simulink model "Basic_DMT"  (R2014b)
settings: Solver=FixedStepDiscrete  SolverMode=SingleTasking  StartTime=0.0  StopTime=25e-6-14e-9*24  RelTol=1e-3
PreLoadFcn:
  | userName = getenv('UserName');
  | 
  | if strcmp(userName,'Tim')
  | cd C:\Users\Tim\Documents\GitHub\MA_1\Basic_DMT
  | else
  | cd C:\Users\Tim-UML\Documents\GitHub\MA_1\Basic_DMT
  | end
InitFcn:
  | userName = getenv('UserName');
  | 
  | if strcmp(userName,'Tim')
  | cd C:\Users\Tim\Documents\GitHub\MA_1\Basic_DMT
  | else
  | cd C:\Users\Tim-UML\Documents\GitHub\MA_1\Basic_DMT
  | end
values from neighbouring files (symbols this model uses):
  a0 = 0.21194908595403703    (= 0.211949085954)    [initScript.m]
  a1 = 0.576101828091926    (= 0.576101828092)    [initScript.m]
  a2 = a0    (= 0.211949085954)    [initScript.m]
  beta = 1    [initScript.m]
  bitPerSymb = 4    [initScript.m]
  chanDownFact = Tchan/SystemPeriod    [initScript.m]
  fftLen = 16    [initScript.m]
  fftLenActive = fftLenDMT    (= 32)    [initScript.m]
  fftLenDMT = 2*fftLen    (= 32)    [initScript.m]
  GI_Active = GI_LenDMT    (= 0)    [initScript.m]
  GI_Len = 0    [initScript.m]
  GI_LenDMT = 0    [initScript.m]
  M = log2(fftLen)    [initScript.m]
  sysgenSystemPeriod = 4e-9    (= 4e-09)    [initScript.m]
  SystemPeriod = 4e-9    (= 4e-09)    [initScript.m]
  upsampleFactor = 1    [initScript.m]
  usedSubCar = 14    [initScript.m]
undefined symbols (not defined in the file or in its folder): bitCount, get, modu_mode, Tb, Ts
libraries: xbsIndex_r4 x822, commdigbbndam3 x59, simulink x42, dspsigops x7, commrandsrc2 x6, dspbuff3 x4, dspxfrm3 x3, dspswit3 x2, commseqgen2 x1, dsparch4 x1, commutil2 x1, dspsnks4 x1
(part 4 of 10)

== system Basic_DMT/Demodulation/Bit Demapping P11 ==
  mode : Inport
  data : Inport  Port=2
  16-QAM : Subsystem
  256-QAM : Subsystem
  Fcn : Fcn  Expr=u==0
  Fcn1 : Fcn  Expr=u==1
  Merge : Merge
  Out1 : Outport
  wires:
  data/1 -> 16-QAM/1(In1), 256-QAM/1(In1)
  Fcn/1 -> 256-QAM/Enable
  mode/1 -> Fcn1/1, Fcn/1
  Merge/1 -> Out1/1
  Fcn1/1 -> 16-QAM/Enable
  256-QAM/1(Out1) -> Merge/2
  16-QAM/1(Out1) -> Merge/1

== system Basic_DMT/Demodulation/Bit Demapping P12 ==
  mode : Inport
  data : Inport  Port=2
  16-QAM : Subsystem
  256-QAM : Subsystem
  Fcn : Fcn  Expr=u==0
  Fcn1 : Fcn  Expr=u==1
  Merge : Merge
  Out1 : Outport
  wires:
  data/1 -> 16-QAM/1(In1), 256-QAM/1(In1)
  Fcn/1 -> 256-QAM/Enable
  mode/1 -> Fcn1/1, Fcn/1
  Merge/1 -> Out1/1
  Fcn1/1 -> 16-QAM/Enable
  256-QAM/1(Out1) -> Merge/2
  16-QAM/1(Out1) -> Merge/1

== system Basic_DMT/Demodulation/Bit Demapping P13 ==
  mode : Inport
  data : Inport  Port=2
  16-QAM : Subsystem
  256-QAM : Subsystem
  Fcn : Fcn  Expr=u==0
  Fcn1 : Fcn  Expr=u==1
  Merge : Merge
  Out1 : Outport
  wires:
  data/1 -> 16-QAM/1(In1), 256-QAM/1(In1)
  Fcn/1 -> 256-QAM/Enable
  mode/1 -> Fcn1/1, Fcn/1
  Merge/1 -> Out1/1
  Fcn1/1 -> 16-QAM/Enable
  256-QAM/1(Out1) -> Merge/2
  16-QAM/1(Out1) -> Merge/1

== system Basic_DMT/Demodulation/Bit Demapping P14 ==
  mode : Inport
  data : Inport  Port=2
  16-QAM : Subsystem
  256-QAM : Subsystem
  Fcn : Fcn  Expr=u==0
  Fcn1 : Fcn  Expr=u==1
  Merge : Merge
  Out1 : Outport
  wires:
  data/1 -> 16-QAM/1(In1), 256-QAM/1(In1)
  Fcn/1 -> 256-QAM/Enable
  mode/1 -> Fcn1/1, Fcn/1
  Merge/1 -> Out1/1
  Fcn1/1 -> 16-QAM/Enable
  256-QAM/1(Out1) -> Merge/2
  16-QAM/1(Out1) -> Merge/1

== system Basic_DMT/Demodulation/Bit Demapping P2 ==
  mode : Inport
  data : Inport  Port=2
  16-QAM : Subsystem
  256-QAM : Subsystem
  Fcn : Fcn  Expr=u==0
  Fcn1 : Fcn  Expr=u==1
  Merge : Merge
  Out1 : Outport
  wires:
  data/1 -> 16-QAM/1(In1), 256-QAM/1(In1)
  Fcn/1 -> 256-QAM/Enable
  mode/1 -> Fcn1/1, Fcn/1
  Merge/1 -> Out1/1
  Fcn1/1 -> 16-QAM/Enable
  256-QAM/1(Out1) -> Merge/2
  16-QAM/1(Out1) -> Merge/1

== system Basic_DMT/Demodulation/Bit Demapping P3 ==
  mode : Inport
  data : Inport  Port=2
  16-QAM : Subsystem
  256-QAM : Subsystem
  Fcn : Fcn  Expr=u==0
  Fcn1 : Fcn  Expr=u==1
  Merge : Merge
  Out1 : Outport
  wires:
  data/1 -> 16-QAM/1(In1), 256-QAM/1(In1)
  Fcn/1 -> 256-QAM/Enable
  mode/1 -> Fcn1/1, Fcn/1
  Merge/1 -> Out1/1
  Fcn1/1 -> 16-QAM/Enable
  256-QAM/1(Out1) -> Merge/2
  16-QAM/1(Out1) -> Merge/1

== system Basic_DMT/Demodulation/Bit Demapping P4 ==
  mode : Inport
  data : Inport  Port=2
  16-QAM : Subsystem
  256-QAM : Subsystem
  Fcn : Fcn  Expr=u==0
  Fcn1 : Fcn  Expr=u==1
  Merge : Merge
  Out1 : Outport
  wires:
  data/1 -> 16-QAM/1(In1), 256-QAM/1(In1)
  Fcn/1 -> 256-QAM/Enable
  mode/1 -> Fcn1/1, Fcn/1
  Merge/1 -> Out1/1
  Fcn1/1 -> 16-QAM/Enable
  256-QAM/1(Out1) -> Merge/2
  16-QAM/1(Out1) -> Merge/1

== system Basic_DMT/Demodulation/Bit Demapping P5 ==
  mode : Inport
  data : Inport  Port=2
  16-QAM : Subsystem
  256-QAM : Subsystem
  Fcn : Fcn  Expr=u==0
  Fcn1 : Fcn  Expr=u==1
  Merge : Merge
  Out1 : Outport
  wires:
  data/1 -> 16-QAM/1(In1), 256-QAM/1(In1)
  Fcn/1 -> 256-QAM/Enable
  mode/1 -> Fcn1/1, Fcn/1
  Merge/1 -> Out1/1
  Fcn1/1 -> 16-QAM/Enable
  256-QAM/1(Out1) -> Merge/2
  16-QAM/1(Out1) -> Merge/1

== system Basic_DMT/Demodulation/Bit Demapping P6 ==
  mode : Inport
  data : Inport  Port=2
  16-QAM : Subsystem
  256-QAM : Subsystem
  Fcn : Fcn  Expr=u==0
  Fcn1 : Fcn  Expr=u==1
  Merge : Merge
  Out1 : Outport
  wires:
  data/1 -> 16-QAM/1(In1), 256-QAM/1(In1)
  Fcn/1 -> 256-QAM/Enable
  mode/1 -> Fcn1/1, Fcn/1
  Merge/1 -> Out1/1
  Fcn1/1 -> 16-QAM/Enable
  256-QAM/1(Out1) -> Merge/2
  16-QAM/1(Out1) -> Merge/1

== system Basic_DMT/Demodulation/Bit Demapping P7 ==
  mode : Inport
  data : Inport  Port=2
  16-QAM : Subsystem
  256-QAM : Subsystem
  Fcn : Fcn  Expr=u==0
  Fcn1 : Fcn  Expr=u==1
  Merge : Merge
  Out1 : Outport
  wires:
  data/1 -> 16-QAM/1(In1), 256-QAM/1(In1)
  Fcn/1 -> 256-QAM/Enable
  mode/1 -> Fcn1/1, Fcn/1
  Merge/1 -> Out1/1
  Fcn1/1 -> 16-QAM/Enable
  256-QAM/1(Out1) -> Merge/2
  16-QAM/1(Out1) -> Merge/1

== system Basic_DMT/Demodulation/Bit Demapping P8 ==
  mode : Inport
  data : Inport  Port=2
  16-QAM : Subsystem
  256-QAM : Subsystem
  Fcn : Fcn  Expr=u==0
  Fcn1 : Fcn  Expr=u==1
  Merge : Merge
  Out1 : Outport
  wires:
  data/1 -> 16-QAM/1(In1), 256-QAM/1(In1)
  Fcn/1 -> 256-QAM/Enable
  mode/1 -> Fcn1/1, Fcn/1
  Merge/1 -> Out1/1
  Fcn1/1 -> 16-QAM/Enable
  256-QAM/1(Out1) -> Merge/2
  16-QAM/1(Out1) -> Merge/1

== system Basic_DMT/Demodulation/Bit Demapping P9 ==
  mode : Inport
  data : Inport  Port=2
  16-QAM : Subsystem
  256-QAM : Subsystem
  Fcn : Fcn  Expr=u==0
  Fcn1 : Fcn  Expr=u==1
  Merge : Merge
  Out1 : Outport
  wires:
  data/1 -> 16-QAM/1(In1), 256-QAM/1(In1)
  Fcn/1 -> 256-QAM/Enable
  mode/1 -> Fcn1/1, Fcn/1
  Merge/1 -> Out1/1
  Fcn1/1 -> 16-QAM/Enable
  256-QAM/1(Out1) -> Merge/2
  16-QAM/1(Out1) -> Merge/1

== system Basic_DMT/IFFTaPIS/Assert_After_Create_Frame ==
  In1 : Inport
  In2 : Inport  Port=2
  In3 : Inport  Port=3
  Add1 : Sum  Inputs=+-
  Add3 : Sum  Inputs=+-
  Check Static Range1 : simulink/Model Verification/Check  Static Range  Description=0 <= u <= 0  max=0  max_included=on  min=0  min_included=on  enabled=on  stopWhenAssertionFail=off  export=off  icon=graphic
  Check Static Range3 : simulink/Model Verification/Check  Static Range  Description=0 <= u <= 0  max=0  max_included=on  min=0  min_included=on  enabled=on  stopWhenAssertionFail=off  export=off  icon=graphic
  Complex to Real-Imag : ComplexToRealImag
  Delay : Delay  DelayLength=1  InitialCondition=0
  Gateway Out6 : xbsIndex_r4/Gateway Out  inherit_from_input=off  hdl_port=off  rows=1  columns=1  UseAsDAC=off  DACChannel='1'  interface=None  automatic_assignment=on  address_offset=hex2dec('00')  intf_description=''  timing_constraint=None  locs_specified=off  LOCs={}  io_standard={}  block_type=gatewayout
  Gateway Out7 : xbsIndex_r4/Gateway Out  inherit_from_input=off  hdl_port=off  rows=1  columns=1  UseAsDAC=off  DACChannel='1'  interface=None  automatic_assignment=on  address_offset=hex2dec('00')  intf_description=''  timing_constraint=None  locs_specified=off  LOCs={}  io_standard={}  block_type=gatewayout
  Scope1 : Scope  NumInputPorts=6
      settings: TimeRange=4.014342186534899e-07  YMin=-3~-3~-4~-4~-4~-10  YMax=1~1~4~4~4~10  SaveName=ScopeData24
  Unbuffer2 : Unbuffer  SampleBasedProcessing=Same as frame based
  wires:
  In2/1 -> Gateway Out6/1
  In3/1 -> Gateway Out7/1
  Complex to Real-Imag/1 -> Scope1/1, Add3/1
  Gateway Out6/1 -> Scope1/2, Add3/2
  Add3/1 -> Scope1/3, Check Static Range3/1
  Gateway Out7/1 -> Scope1/5, Add1/2
  Complex to Real-Imag/2 -> Scope1/4, Add1/1
  Add1/1 -> Scope1/6, Check Static Range1/1
  Unbuffer2/1 -> Delay/1
  Delay/1 -> Complex to Real-Imag/1
  In1/1 -> Unbuffer2/1

== system Basic_DMT/IFFTaPIS/Assert_After_IFFT ==
  In1 : Inport
  In2 : Inport  Port=2
  In3 : Inport  Port=3
  Add1 : Sum  Inputs=+-
  Add3 : Sum  Inputs=+-
  Check Static Range1 : simulink/Model Verification/Check  Static Range  Description=0 <= u <= 0  max=0  max_included=on  min=0  min_included=on  enabled=on  stopWhenAssertionFail=off  export=off  icon=graphic
  Check Static Range3 : simulink/Model Verification/Check  Static Range  Description=0 <= u <= 0  max=0  max_included=on  min=0  min_included=on  enabled=on  stopWhenAssertionFail=off  export=off  icon=graphic
  Complex to Real-Imag : ComplexToRealImag
  Delay : Delay  Commented=through  DelayLength=1  InitialCondition=0
  Gateway Out6 : xbsIndex_r4/Gateway Out  inherit_from_input=off  hdl_port=off  rows=1  columns=1  UseAsDAC=off  DACChannel='1'  interface=None  automatic_assignment=on  address_offset=hex2dec('00')  intf_description=''  timing_constraint=None  locs_specified=off  LOCs={}  io_standard={}  block_type=gatewayout
  Gateway Out7 : xbsIndex_r4/Gateway Out  inherit_from_input=off  hdl_port=off  rows=1  columns=1  UseAsDAC=off  DACChannel='1'  interface=None  automatic_assignment=on  address_offset=hex2dec('00')  intf_description=''  timing_constraint=None  locs_specified=off  LOCs={}  io_standard={}  block_type=gatewayout
  Scope1 : Scope  NumInputPorts=6
      settings: YMin=-5~-5~-5~-5~-5~-5  YMax=5~5~5~5~5~5  SaveName=ScopeData24
  Unbuffer2 : Unbuffer  SampleBasedProcessing=Same as frame based
  wires:
  In2/1 -> Gateway Out6/1
  In3/1 -> Gateway Out7/1
  Complex to Real-Imag/1 -> Scope1/1, Add3/1
  Gateway Out6/1 -> Add3/2, Scope1/2
  Add3/1 -> Check Static Range3/1, Scope1/3
  Gateway Out7/1 -> Add1/2, Scope1/5
  Complex to Real-Imag/2 -> Add1/1, Scope1/4
  Add1/1 -> Check Static Range1/1, Scope1/6
  Unbuffer2/1 -> Delay/1
  Delay/1 -> Complex to Real-Imag/1
  In1/1 -> Unbuffer2/1

== system Basic_DMT/IFFTaPIS/Assert_aft_GI ==
  In1 : Inport
  In2 : Inport  Port=2
  In3 : Inport  Port=3
  Abs{,1..5} (6 alike) : Abs
  Add1 : Sum  Inputs=+-
  Add2 : Sum  Inputs=+-
  Add3 : Sum  Inputs=+-
  Complex to Real-Imag : ComplexToRealImag
  Data Type Conversion1 : DataTypeConversion  OutDataTypeStr=double
  Data Type Conversion2 : DataTypeConversion  OutDataTypeStr=double
  Delay : Delay  Commented=through  DelayLength=62  InitialCondition=0
  Divide : Product  Inputs=*/
  Divide1 : Product  Inputs=*/
  Divide2 : Product  Inputs=*/
  Gateway Out6 : xbsIndex_r4/Gateway Out  inherit_from_input=off  hdl_port=off  rows=1  columns=1  UseAsDAC=off  DACChannel='1'  interface=None  automatic_assignment=on  address_offset=hex2dec('00')  intf_description=''  timing_constraint=None  locs_specified=off  LOCs={}  io_standard={}  block_type=gatewayout
  Gateway Out7 : xbsIndex_r4/Gateway Out  inherit_from_input=off  hdl_port=off  rows=1  columns=1  UseAsDAC=off  DACChannel='1'  interface=None  automatic_assignment=on  address_offset=hex2dec('00')  intf_description=''  timing_constraint=None  locs_specified=off  LOCs={}  io_standard={}  block_type=gatewayout
  MinMax : MinMax  Function=max  Inputs=2
  MinMax1 : MinMax  Function=max  Inputs=2
  MinMax2 : MinMax  Function=max  Inputs=2
  Real-Imag to Complex : RealImagToComplex
  Scope1 : Scope  Commented=on  NumInputPorts=4
      settings: YMin=-5~-5~-5~-5  YMax=5~5~5~5  SaveName=ScopeData23
  Scope10 : Scope  NumInputPorts=4
      settings: TimeRange=5e-05  YMin=-5~-5~-5~-5  YMax=5~5~5~5  SaveName=ScopeData20
  Scope3 : Scope  Commented=on  NumInputPorts=4
      settings: TimeRange=5e-05  YMin=-5~-5~-5~-5  YMax=5~5~5~5  SaveName=ScopeData21
  wires:
  Data Type Conversion2/1 -> Abs1/1
  Add1/1 -> Scope10/3, Divide/1
  In1/1 -> Delay/1
  Complex to Real-Imag/1 -> Add1/1, Abs3/1, Scope10/1
  In3/1 -> Gateway Out7/1
  In2/1 -> Gateway Out6/1
  Abs/1 -> MinMax2/2, Add3/2, Scope1/2
  Add3/1 -> Divide2/1, Scope1/3
  Abs1/1 -> Scope1/1, MinMax2/1, Add3/1
  Gateway Out6/1 -> Real-Imag to Complex/1, Add1/2, Abs2/1, Scope10/2
  Data Type Conversion1/1 -> Abs/1
  Real-Imag to Complex/1 -> Data Type Conversion1/1
  Delay/1 -> Data Type Conversion2/1, Complex to Real-Imag/1
  MinMax/1 -> Divide/2
  Divide/1 -> Scope10/4
  Add2/1 -> Divide1/1, Scope3/3
  Complex to Real-Imag/2 -> Abs4/1, Scope3/1, Add2/1
  Gateway Out7/1 -> Real-Imag to Complex/2, Abs5/1, Scope3/2, Add2/2
  MinMax1/1 -> Divide1/2
  Divide1/1 -> Scope3/4
  Divide2/1 -> Scope1/4
  MinMax2/1 -> Divide2/2
  Abs2/1 -> MinMax/2
  Abs3/1 -> MinMax/1
  Abs4/1 -> MinMax1/1
  Abs5/1 -> MinMax1/2

== system Basic_DMT/IFFTaPIS/Create_Frame_for_IFFT ==
  note: Unbuffer necessary,
      |  because of frame based signal
  Sub1 : Inport
  Sub2 : Inport  Port=2
  Sub3 : Inport  Port=3
  Sub4 : Inport  Port=4
  Sub5 : Inport  Port=5
  Sub6 : Inport  Port=6
  Sub7 : Inport  Port=7
  Sub8 : Inport  Port=8
  Sub9 : Inport  Port=9
  Sub10 : Inport  Port=10
  Sub11 : Inport  Port=11
  Sub12 : Inport  Port=12
  Sub13 : Inport  Port=13
  Sub14 : Inport  Port=14
  OFDMorDMT : Subsystem  Variant=on
  Unbuffer{1..14} (14 alike) : Unbuffer  SampleBasedProcessing=Same as frame based
  Out1 : Outport
  wires:
  Sub2/1 -> Unbuffer2/1
  Sub1/1 -> Unbuffer3/1
  Unbuffer2/1 -> OFDMorDMT/2(Sub2)
  Unbuffer3/1 -> OFDMorDMT/1(Sub1)
  OFDMorDMT/1(Out1) -> Out1/1
  Sub4/1 -> Unbuffer1/1
  Sub3/1 -> Unbuffer4/1
  Unbuffer1/1 -> OFDMorDMT/4(Sub4)
  Unbuffer4/1 -> OFDMorDMT/3(Sub3)
  Sub6/1 -> Unbuffer5/1
  Sub5/1 -> Unbuffer6/1
  Unbuffer5/1 -> OFDMorDMT/6(Sub6)
  Unbuffer6/1 -> OFDMorDMT/5(Sub5)
  Sub8/1 -> Unbuffer7/1
  Sub7/1 -> Unbuffer8/1
  Unbuffer7/1 -> OFDMorDMT/8(Sub8)
  Unbuffer8/1 -> OFDMorDMT/7(Sub7)
  Sub10/1 -> Unbuffer9/1
  Sub9/1 -> Unbuffer10/1
  Unbuffer9/1 -> OFDMorDMT/10(Sub10)
  Unbuffer10/1 -> OFDMorDMT/9(Sub9)
  Sub11/1 -> Unbuffer11/1
  Unbuffer11/1 -> OFDMorDMT/11(Sub11)
  Sub13/1 -> Unbuffer14/1
  Unbuffer14/1 -> OFDMorDMT/13(Sub13)
  Sub14/1 -> Unbuffer13/1
  Unbuffer13/1 -> OFDMorDMT/14(Sub14)
  Sub12/1 -> Unbuffer12/1
  Unbuffer12/1 -> OFDMorDMT/12(Sub12)

== system Basic_DMT/IFFTaPIS/FSM_FIFO ==
  In1 : Inport  SampleTime=bitPerSymb*usedSubCar*SystemPeriod
  Buffer : Buffer  N=fftLenActive  TreatMby1Signals=One channel
  Complex to Real-Imag{,1..3} (4 alike) : ComplexToRealImag
  Constant2 : Constant  Value=0  SampleTime=SystemPeriod
  Data Store Memory3 : DataStoreMemory  DataStoreName=state  OutDataTypeStr=double
  Data Store Memory4 : DataStoreMemory  DataStoreName=k  OutDataTypeStr=double
  Data Store Memory5 : DataStoreMemory  DataStoreName=loopCount  OutDataTypeStr=double
  Delay : Delay  DelayLength=1  InitialCondition=0
  Index Vector : MultiPortSwitch  DataPortOrder=Zero-based contiguous  Inputs=2  zeroidx=on
  MATLAB Function1 : MATLAB Function  TreatAsAtomicUnit=on  SystemSampleTime=SystemPeriod
  Queue1 : dspbuff3/Queue  depth=64  trigger=Non-zero sample  overflow=Dynamic reallocation  pes=Warning  eso=off  fso=off  nso=on  clr=off  clrOutport=off  adf=off
  Real-Imag to Complex1 : RealImagToComplex
  Scope : Scope  NumInputPorts=2
      settings: YMin=-5~-5  YMax=5~5  SaveName=ScopeData77
  Scope1 : Scope  NumInputPorts=2
      settings: YMin=-5~-5  YMax=5~5  SaveName=ScopeData78
  Unbuffer1 : Unbuffer  ic=64e-9  SampleBasedProcessing=Same as frame based
  Unbuffer2 : Unbuffer  ic=64e-9  SampleBasedProcessing=Same as frame based
  Zero-Order Hold : ZeroOrderHold  SampleTime=SystemPeriod
  Zero-Order Hold1 : ZeroOrderHold  SampleTime=SystemPeriod*16
  Out1 : Outport
  wires:
  Index Vector/1 -> Buffer/1
  MATLAB Function1/3(pop) -> Queue1/3
  MATLAB Function1/2(push) -> Queue1/2
  Constant2/1 -> Real-Imag to Complex1/2, Real-Imag to Complex1/1
  Delay/1 -> MATLAB Function1/1(num)
  MATLAB Function1/1(sel) -> Index Vector/1
  Queue1/1 -> Index Vector/3
  Real-Imag to Complex1/1 -> Index Vector/2
  Buffer/1 -> Out1/1
  Queue1/2 -> Delay/1
  Zero-Order Hold/1 -> Complex to Real-Imag1/1, Queue1/1
  Unbuffer2/1 -> Complex to Real-Imag2/1, Complex to Real-Imag/1, Zero-Order Hold/1
  Complex to Real-Imag/1 -> Scope/1
  Complex to Real-Imag1/1 -> Scope/2
  Zero-Order Hold1/1 -> Unbuffer1/1
  Unbuffer1/1 -> Complex to Real-Imag3/1
  In1/1 -> Zero-Order Hold1/1, Unbuffer2/1
  Complex to Real-Imag2/1 -> Scope1/1
  Complex to Real-Imag3/1 -> Scope1/2

== system Basic_DMT/IFFTaPIS/Guard_Interval ==
  note: 1) Add Subsystem or Model blocks as valid variant choices.
      | 2) You cannot connect blocks at this level. At simulation, connectivity is automatically
      | determined, based on the active variant and port name matching.
  In1 : Inport
  None : Subsystem  VariantControl=guardInterval==1
  Set_GI_DMT : Subsystem  VariantControl=guardInterval==2&&dmtOfdm==2
  Set_GI_OFDM : Subsystem  VariantControl=guardInterval==2&&dmtOfdm==1
  Out1 : Outport
  pop : Outport  Port=2

== system Basic_DMT/IFFTaPIS/upsample ==
  note: 1) Add Subsystem or Model blocks as valid variant choices.
      | 2) You cannot connect blocks at this level. At simulation, connectivity is automatically
      | determined, based on the active variant and port name matching.
  In1 : Inport
  upsample_No : Subsystem  VariantControl=upsample==1
  upsample_yes : Subsystem  VariantControl=upsample==2
  Out1 : Outport

== system Basic_DMT/Modulation/Assert_aft_Mapping ==
  Sub1 : Inport
  Sub2 : Inport  Port=2
  sg_sub1_re : Inport  Port=3
  sg_sub1_im : Inport  Port=4
  sg_sub2_re : Inport  Port=5
  sg_sub2_im : Inport  Port=6
  Add{1..4} (4 alike) : Sum  Inputs=+-
  Check Static Range{1..4} (4 alike) : simulink/Model Verification/Check  Static Range  Description=0 <= u <= 0  max=0  max_included=on  min=0  min_included=on  enabled=on  stopWhenAssertionFail=off  export=off  icon=graphic
  Complex to Real-Imag : ComplexToRealImag
  Complex to Real-Imag1 : ComplexToRealImag
  Gateway Out{1..2,6..7} (4 alike) : xbsIndex_r4/Gateway Out  inherit_from_input=off  hdl_port=off  rows=1  columns=1  UseAsDAC=off  DACChannel='1'  interface=None  automatic_assignment=on  address_offset=hex2dec('00')  intf_description=''  timing_constraint=None  locs_specified=off  LOCs={}  io_standard={}  block_type=gatewayout
  Scope{1..3,10} (4 alike) : Scope  Commented=on  NumInputPorts=3
      Scope1 settings: YMin=-5~-5~-5  YMax=5~5~5  SaveName=ScopeData25
      Scope10 settings: YMin=-5~-5~-5  YMax=5~5~5  SaveName=ScopeData14
      Scope2 settings: YMin=-5~-5~-5  YMax=5~5~5  SaveName=ScopeData26
      Scope3 settings: YMin=-5~-5~-5  YMax=5~5~5  SaveName=ScopeData8
  wires:
  Gateway Out7/1 -> Scope3/2, Add2/2
  Add1/1 -> Check Static Range2/1, Scope10/3
  Gateway Out6/1 -> Scope10/2, Add1/2
  Complex to Real-Imag/2 -> Scope3/1, Add2/1
  Complex to Real-Imag/1 -> Add1/1, Scope10/1
  Sub1/1 -> Complex to Real-Imag/1
  Add2/1 -> Check Static Range1/1, Scope3/3
  sg_sub1_re/1 -> Gateway Out6/1
  sg_sub1_im/1 -> Gateway Out7/1
  sg_sub2_re/1 -> Gateway Out1/1
  sg_sub2_im/1 -> Gateway Out2/1
  Gateway Out2/1 -> Scope2/2, Add4/2
  Add3/1 -> Check Static Range4/1, Scope1/3
  Gateway Out1/1 -> Scope1/2, Add3/2
  Complex to Real-Imag1/2 -> Scope2/1, Add4/1
  Complex to Real-Imag1/1 -> Add3/1, Scope1/1
  Add4/1 -> Check Static Range3/1, Scope2/3
  Sub2/1 -> Complex to Real-Imag1/1

== system Basic_DMT/Modulation/Bit_Mapping_P1 ==
  mode : Inport
  data : Inport  Port=2
  16_QAM : Subsystem
  256_QAM : Subsystem  RequirementInfo="{}  %GIDa_05459083_aa94_49a4_b754_f58c2abee340"
  Fcn : Fcn  Expr=u==0
  Fcn1 : Fcn  Expr=u==1
  Merge : Merge
  Out1 : Outport
  wires:
  Fcn/1 -> 256_QAM/Enable
  mode/1 -> Fcn1/1, Fcn/1
  Merge/1 -> Out1/1
  256_QAM/1(Out1) -> Merge/2
  Fcn1/1 -> 16_QAM/Enable
  16_QAM/1(Out1) -> Merge/1
  data/1 -> 16_QAM/1(In1), 256_QAM/1(In1)

== system Basic_DMT/Modulation/Bit_Mapping_P10 ==
  mode : Inport
  data : Inport  Port=2
  16_QAM : Subsystem
  256_QAM : Subsystem  RequirementInfo={} %GIDa_af48e1d8_7483_434c_820c_a1ec0e5e1719
  Fcn : Fcn  Expr=u==0
  Fcn1 : Fcn  Expr=u==1
  Merge : Merge
  Out1 : Outport
  wires:
  Fcn/1 -> 256_QAM/Enable
  mode/1 -> Fcn1/1, Fcn/1
  Merge/1 -> Out1/1
  256_QAM/1(Out1) -> Merge/2
  Fcn1/1 -> 16_QAM/Enable
  16_QAM/1(Out1) -> Merge/1
  data/1 -> 16_QAM/1(In1), 256_QAM/1(In1)

== system Basic_DMT/Modulation/Bit_Mapping_P11 ==
  mode : Inport
  data : Inport  Port=2
  16_QAM : Subsystem
  256_QAM : Subsystem  RequirementInfo={} %GIDa_3309a449_da50_4542_90e7_11734bda5c39
  Fcn : Fcn  Expr=u==0
  Fcn1 : Fcn  Expr=u==1
  Merge : Merge
  Out1 : Outport
  wires:
  Fcn/1 -> 256_QAM/Enable
  mode/1 -> Fcn1/1, Fcn/1
  Merge/1 -> Out1/1
  256_QAM/1(Out1) -> Merge/2
  Fcn1/1 -> 16_QAM/Enable
  16_QAM/1(Out1) -> Merge/1
  data/1 -> 16_QAM/1(In1), 256_QAM/1(In1)

== system Basic_DMT/Modulation/Bit_Mapping_P12 ==
  mode : Inport
  data : Inport  Port=2
  16_QAM : Subsystem
  256_QAM : Subsystem  RequirementInfo={} %GIDa_17b76de1_447f_4e1d_a5cb_350e5302a50c
  Fcn : Fcn  Expr=u==0
  Fcn1 : Fcn  Expr=u==1
  Merge : Merge
  Out1 : Outport
  wires:
  Fcn/1 -> 256_QAM/Enable
  mode/1 -> Fcn1/1, Fcn/1
  Merge/1 -> Out1/1
  256_QAM/1(Out1) -> Merge/2
  Fcn1/1 -> 16_QAM/Enable
  16_QAM/1(Out1) -> Merge/1
  data/1 -> 16_QAM/1(In1), 256_QAM/1(In1)

== system Basic_DMT/Modulation/Bit_Mapping_P13 ==
  mode : Inport
  data : Inport  Port=2
  16_QAM : Subsystem
  256_QAM : Subsystem  RequirementInfo={} %GIDa_f14c61b1_d51c_481e_b1a8_5d3d4ac2a9e9
  Fcn : Fcn  Expr=u==0
  Fcn1 : Fcn  Expr=u==1
  Merge : Merge
  Out1 : Outport
  wires:
  Fcn/1 -> 256_QAM/Enable
  mode/1 -> Fcn1/1, Fcn/1
  Merge/1 -> Out1/1
  256_QAM/1(Out1) -> Merge/2
  Fcn1/1 -> 16_QAM/Enable
  16_QAM/1(Out1) -> Merge/1
  data/1 -> 16_QAM/1(In1), 256_QAM/1(In1)

== system Basic_DMT/Modulation/Bit_Mapping_P14 ==
  mode : Inport
  data : Inport  Port=2
  16_QAM : Subsystem
  256_QAM : Subsystem  RequirementInfo={} %GIDa_5a820fc7_0f9e_48f0_a6bb_13204884edc3
  Fcn : Fcn  Expr=u==0
  Fcn1 : Fcn  Expr=u==1
  Merge : Merge
  Out1 : Outport
  wires:
  Fcn/1 -> 256_QAM/Enable
  mode/1 -> Fcn1/1, Fcn/1
  Merge/1 -> Out1/1
  256_QAM/1(Out1) -> Merge/2
  Fcn1/1 -> 16_QAM/Enable
  16_QAM/1(Out1) -> Merge/1
  data/1 -> 16_QAM/1(In1), 256_QAM/1(In1)

== system Basic_DMT/Modulation/Bit_Mapping_P2 ==
  mode : Inport
  data : Inport  Port=2
  16_QAM : Subsystem
  256_QAM : Subsystem  RequirementInfo={} %GIDa_18f84a92_91ee_4bad_9239_e5fa1d23e11f
  Fcn : Fcn  Expr=u==0
  Fcn1 : Fcn  Expr=u==1
  Merge : Merge
  Out1 : Outport
  wires:
  Fcn/1 -> 256_QAM/Enable
  mode/1 -> Fcn1/1, Fcn/1
  Merge/1 -> Out1/1
  256_QAM/1(Out1) -> Merge/2
  Fcn1/1 -> 16_QAM/Enable
  16_QAM/1(Out1) -> Merge/1
  data/1 -> 16_QAM/1(In1), 256_QAM/1(In1)

== system Basic_DMT/Modulation/Bit_Mapping_P3 ==
  mode : Inport
  data : Inport  Port=2
  16_QAM : Subsystem
  256_QAM : Subsystem  RequirementInfo={} %GIDa_b2d0a792_063c_4424_a28d_b377e68cb813
  Fcn : Fcn  Expr=u==0
  Fcn1 : Fcn  Expr=u==1
  Merge : Merge
  Out1 : Outport
  wires:
  Fcn/1 -> 256_QAM/Enable
  mode/1 -> Fcn1/1, Fcn/1
  Merge/1 -> Out1/1
  256_QAM/1(Out1) -> Merge/2
  Fcn1/1 -> 16_QAM/Enable
  16_QAM/1(Out1) -> Merge/1
  data/1 -> 16_QAM/1(In1), 256_QAM/1(In1)

== system Basic_DMT/Modulation/Bit_Mapping_P4 ==
  mode : Inport
  data : Inport  Port=2
  16_QAM : Subsystem
  256_QAM : Subsystem  RequirementInfo={} %GIDa_e32f567a_13bc_4104_a0e4_62a916a72463
  Fcn : Fcn  Expr=u==0
  Fcn1 : Fcn  Expr=u==1
  Merge : Merge
  Out1 : Outport
  wires:
  Fcn/1 -> 256_QAM/Enable
  mode/1 -> Fcn1/1, Fcn/1
  Merge/1 -> Out1/1
  256_QAM/1(Out1) -> Merge/2
  Fcn1/1 -> 16_QAM/Enable
  16_QAM/1(Out1) -> Merge/1
  data/1 -> 16_QAM/1(In1), 256_QAM/1(In1)

== system Basic_DMT/Modulation/Bit_Mapping_P5 ==
  mode : Inport
  data : Inport  Port=2
  16_QAM : Subsystem
  256_QAM : Subsystem  RequirementInfo={} %GIDa_02e65cfb_927d_410f_9407_7314ebe98b6e
  Fcn : Fcn  Expr=u==0
  Fcn1 : Fcn  Expr=u==1
  Merge : Merge
  Out1 : Outport
  wires:
  Fcn/1 -> 256_QAM/Enable
  mode/1 -> Fcn1/1, Fcn/1
  Merge/1 -> Out1/1
  256_QAM/1(Out1) -> Merge/2
  Fcn1/1 -> 16_QAM/Enable
  16_QAM/1(Out1) -> Merge/1
  data/1 -> 16_QAM/1(In1), 256_QAM/1(In1)

== system Basic_DMT/Modulation/Bit_Mapping_P6 ==
  mode : Inport
  data : Inport  Port=2
  16_QAM : Subsystem
  256_QAM : Subsystem  RequirementInfo={} %GIDa_4916751a_a7e0_4ea6_83e2_c37de6ba86c6
  Fcn : Fcn  Expr=u==0
  Fcn1 : Fcn  Expr=u==1
  Merge : Merge
  Out1 : Outport
  wires:
  Fcn/1 -> 256_QAM/Enable
  mode/1 -> Fcn1/1, Fcn/1
  Merge/1 -> Out1/1
  256_QAM/1(Out1) -> Merge/2
  Fcn1/1 -> 16_QAM/Enable
  16_QAM/1(Out1) -> Merge/1
  data/1 -> 16_QAM/1(In1), 256_QAM/1(In1)

== system Basic_DMT/Modulation/Bit_Mapping_P7 ==
  mode : Inport
  data : Inport  Port=2
  16_QAM : Subsystem
  256_QAM : Subsystem  RequirementInfo={} %GIDa_bdb7c520_5a78_4198_9642_f3e58da2ebef
  Fcn : Fcn  Expr=u==0
  Fcn1 : Fcn  Expr=u==1
  Merge : Merge
  Out1 : Outport
  wires:
  Fcn/1 -> 256_QAM/Enable
  mode/1 -> Fcn1/1, Fcn/1
  Merge/1 -> Out1/1
  256_QAM/1(Out1) -> Merge/2
  Fcn1/1 -> 16_QAM/Enable
  16_QAM/1(Out1) -> Merge/1
  data/1 -> 16_QAM/1(In1), 256_QAM/1(In1)

== system Basic_DMT/Modulation/Bit_Mapping_P8 ==
  mode : Inport
  data : Inport  Port=2
  16_QAM : Subsystem
  256_QAM : Subsystem  RequirementInfo={} %GIDa_7182c5e6_6831_4f46_806f_24529648a376
  Fcn : Fcn  Expr=u==0
  Fcn1 : Fcn  Expr=u==1
  Merge : Merge
  Out1 : Outport
  wires:
  Fcn/1 -> 256_QAM/Enable
  mode/1 -> Fcn1/1, Fcn/1
  Merge/1 -> Out1/1
  256_QAM/1(Out1) -> Merge/2
  Fcn1/1 -> 16_QAM/Enable
  16_QAM/1(Out1) -> Merge/1
  data/1 -> 16_QAM/1(In1), 256_QAM/1(In1)

== system Basic_DMT/Modulation/Bit_Mapping_P9 ==
  mode : Inport
  data : Inport  Port=2
  16_QAM : Subsystem
  256_QAM : Subsystem  RequirementInfo={} %GIDa_14494cd8_4714_4206_950b_f7f675e82920
  Fcn : Fcn  Expr=u==0
  Fcn1 : Fcn  Expr=u==1
  Merge : Merge
  Out1 : Outport
  wires:
  Fcn/1 -> 256_QAM/Enable
  mode/1 -> Fcn1/1, Fcn/1
  Merge/1 -> Out1/1
  256_QAM/1(Out1) -> Merge/2
  Fcn1/1 -> 16_QAM/Enable
  16_QAM/1(Out1) -> Merge/1
  data/1 -> 16_QAM/1(In1), 256_QAM/1(In1)

== system Basic_DMT/OFDMorDMT/DMT ==
  In1 : Inport
  remove_GI : Delay  DelayLength=112  InitialCondition=0
  Out1 : Outport
  wires:
  In1/1 -> remove_GI/1
  remove_GI/1 -> Out1/1

== system Basic_DMT/OFDMorDMT/OFDM ==
  In1 : Inport
  Out1 : Outport
  wires:
  In1/1 -> Out1/1

== system Basic_DMT/SIP /Assert DIfferent Output ==
  In1 : Inport
  In2 : Inport  Port=2
  In3 : Inport  Port=3
  In4 : Inport  Port=4
  Add2 : Sum  Inputs=+-
  Add3 : Sum  Inputs=+-
  Check Static Range : simulink/Model Verification/Check  Static Range  Description=0 <= u <= 0  max=0  max_included=on  min=0  min_included=on  enabled=on  stopWhenAssertionFail=off  export=off  icon=graphic
  Check Static Range1 : simulink/Model Verification/Check  Static Range  Description=0 <= u <= 0  max=0  max_included=on  min=0  min_included=on  enabled=on  stopWhenAssertionFail=off  export=off  icon=graphic
  Delay2 : Delay  Commented=through  DelayLength=1  InitialCondition=0  InputProcessing=Columns as channels (frame based)
  Delay3 : Delay  Commented=through  DelayLength=1  InitialCondition=0  InputProcessing=Columns as channels (frame based)
  Gateway Out12 : xbsIndex_r4/Gateway Out  inherit_from_input=on  hdl_port=off  rows=1  columns=1  UseAsDAC=off  DACChannel='1'  interface=None  automatic_assignment=on  address_offset=hex2dec('00')  intf_description=''  timing_constraint=None  locs_specified=off  LOCs={}  io_standard={}  block_type=gatewayout
  Gateway Out13 : xbsIndex_r4/Gateway Out  inherit_from_input=on  hdl_port=off  rows=1  columns=1  UseAsDAC=off  DACChannel='1'  interface=None  automatic_assignment=on  address_offset=hex2dec('00')  intf_description=''  timing_constraint=None  locs_specified=off  LOCs={}  io_standard={}  block_type=gatewayout
  Parallel to Serial : xbsIndex_r4/Parallel to Serial  output_order=Most Significant Word First  arith_type=Unsigned  output_bits=1  bin_pt=0  rst=off  en=off  latency=0  dbl_ovrd=off  block_type=p2s
      settings: infoedit=Each sample presented at the input becomes several samples presented serially at the output.
  Parallel to Serial1 : xbsIndex_r4/Parallel to Serial  output_order=Most Significant Word First  arith_type=Unsigned  output_bits=1  bin_pt=0  rst=off  en=off  latency=0  dbl_ovrd=off  block_type=p2s
      settings: infoedit=Each sample presented at the input becomes several samples presented serially at the output.
  Scope11 : Scope  Commented=on  NumInputPorts=3
      settings: YMin=-5~-5~-5  YMax=5~5~5  SaveName=ScopeData15
  Scope12 : Scope  Commented=on  NumInputPorts=3
      settings: YMin=-5~-5~-5  YMax=5~5~5  SaveName=ScopeData16
  Unbuffer : Unbuffer  SampleBasedProcessing=Same as frame based
  Unbuffer1 : Unbuffer  SampleBasedProcessing=Same as frame based
  wires:
  In4/1 -> Parallel to Serial/1
  Unbuffer1/1 -> Delay3/1
  Delay3/1 -> Add3/1, Scope12/1
  Unbuffer/1 -> Delay2/1
  Add2/1 -> Check Static Range/1, Scope11/3
  Add3/1 -> Check Static Range1/1, Scope12/3
  Parallel to Serial1/1 -> Gateway Out13/1
  Delay2/1 -> Add2/1, Scope11/1
  Gateway Out12/1 -> Add2/2, Scope11/2
  Parallel to Serial/1 -> Gateway Out12/1
  Gateway Out13/1 -> Add3/2, Scope12/2
  In1/1 -> Unbuffer1/1
  In2/1 -> Unbuffer/1
  In3/1 -> Parallel to Serial1/1

== system Basic_DMT/SIPaFFT/Assert_Sub_aft_FFT ==
  sim_DC : Inport
  sim_Sub1 : Inport  Port=2
  sim_Sub2 : Inport  Port=3
  sg_DC_Re : Inport  Port=4
  sg_DC_Im : Inport  Port=5
  sg_Sub1_Re : Inport  Port=6
  sg_Sub1_Im : Inport  Port=7
  sg_Sub2_Re : Inport  Port=8
  sg_Sub2_Im : Inport  Port=9
  Add{1..6} (6 alike) : Sum  Inputs=+-
  Check Static Range{1..6} (6 alike) : simulink/Model Verification/Check  Static Range  Description=-1e-3 <= u <= 1e-3  max=1e-3  max_included=on  min=-1e-3  min_included=on  enabled=on  stopWhenAssertionFail=off  export=off  icon=graphic
  Complex to Real-Imag1 : ComplexToRealImag
  Complex to Real-Imag2 : ComplexToRealImag
  Complex to Real-Imag3 : ComplexToRealImag
  Gateway Out{,1..5} (6 alike) : xbsIndex_r4/Gateway Out  inherit_from_input=on  hdl_port=off  rows=1  columns=1  UseAsDAC=off  DACChannel='1'  interface=None  automatic_assignment=on  address_offset=hex2dec('00')  intf_description=''  timing_constraint=None  locs_specified=off  LOCs={}  io_standard={}  block_type=gatewayout
  Scope1 : Scope  NumInputPorts=6
      settings: TimeRange=7.392000000000001e-05  YMin=2.637524759237758~-4~-2~-0.1983471074380248~-4~-2  YMax=2.716207909295814~4~2~0.7272727272727195~4~2  SaveName=ScopeData11
  Scope2 : Scope  NumInputPorts=6
      settings: YMin=-5~-5~-5~-5~-5~-5  YMax=5~5~5~5~5~5  SaveName=ScopeData27
  Scope3 : Scope  NumInputPorts=6
      settings: YMin=-5~-5~-5~-5~-5~-5  YMax=5~5~5~5~5~5  SaveName=ScopeData28
  wires:
  Add4/1 -> Check Static Range1/1, Scope2/6
  Add2/1 -> Check Static Range3/1, Scope2/3
  sim_DC/1 -> Complex to Real-Imag3/1
  sim_Sub1/1 -> Complex to Real-Imag1/1
  sim_Sub2/1 -> Complex to Real-Imag2/1
  Complex to Real-Imag3/1 -> Scope2/1, Add2/1
  sg_DC_Im/1 -> Gateway Out1/1
  sg_DC_Re/1 -> Gateway Out/1
  Complex to Real-Imag3/2 -> Add4/1, Scope2/4
  Add3/1 -> Check Static Range4/1, Scope1/6
  Add1/1 -> Check Static Range2/1, Scope1/3
  Add6/1 -> Check Static Range6/1, Scope3/6
  Add5/1 -> Check Static Range5/1, Scope3/3
  Complex to Real-Imag1/1 -> Scope1/1, Add1/1
  sg_Sub1_Re/1 -> Gateway Out2/1
  Complex to Real-Imag1/2 -> Add3/1, Scope1/4
  sg_Sub1_Im/1 -> Gateway Out3/1
  Complex to Real-Imag2/1 -> Add5/1, Scope3/1
  sg_Sub2_Re/1 -> Gateway Out4/1
  Complex to Real-Imag2/2 -> Add6/1, Scope3/4
  sg_Sub2_Im/1 -> Gateway Out5/1
  Gateway Out/1 -> Add2/2, Scope2/2
  Gateway Out1/1 -> Add4/2, Scope2/5
  Gateway Out2/1 -> Add1/2, Scope1/2
  Gateway Out3/1 -> Add3/2, Scope1/5
  Gateway Out4/1 -> Scope3/2, Add5/2
  Gateway Out5/1 -> Add6/2, Scope3/5

== system Basic_DMT/SIPaFFT/Assert_aft_DMT ==
  In1 : Inport
  In2 : Inport  Port=2
  In3 : Inport  Port=3
  Add1 : Sum  Inputs=+-
  Add3 : Sum  Inputs=+-
  Check Static Range1 : simulink/Model Verification/Check  Static Range  Description=0 <= u <= 0  max=0  max_included=on  min=0  min_included=on  enabled=on  stopWhenAssertionFail=off  export=off  icon=graphic
  Check Static Range3 : simulink/Model Verification/Check  Static Range  Description=0 <= u <= 0  max=0  max_included=on  min=0  min_included=on  enabled=on  stopWhenAssertionFail=off  export=off  icon=graphic
  Complex to Real-Imag : ComplexToRealImag
  Gateway Out : xbsIndex_r4/Gateway Out  inherit_from_input=on  hdl_port=off  rows=1  columns=1  UseAsDAC=off  DACChannel='1'  interface=None  automatic_assignment=on  address_offset=hex2dec('00')  intf_description=''  timing_constraint=None  locs_specified=off  LOCs={}  io_standard={}  block_type=gatewayout
  Gateway Out1 : xbsIndex_r4/Gateway Out  inherit_from_input=on  hdl_port=off  rows=1  columns=1  UseAsDAC=off  DACChannel='1'  interface=None  automatic_assignment=on  address_offset=hex2dec('00')  intf_description=''  timing_constraint=None  locs_specified=off  LOCs={}  io_standard={}  block_type=gatewayout
  Scope5 : Scope  NumInputPorts=6
      settings: TimeRange=1.34597158739963e-06  YMin=-4~-4~-10~-4~-4~-4  YMax=4~4~10~4~4~4  SaveName=ScopeData18
  Unbuffer : Unbuffer  SampleBasedProcessing=Same as frame based
  wires:
  Complex to Real-Imag/1 -> Scope5/1, Add3/1
  Add3/1 -> Check Static Range3/1, Scope5/3
  Complex to Real-Imag/2 -> Add1/1, Scope5/4
  Add1/1 -> Check Static Range1/1, Scope5/6
  Gateway Out1/1 -> Add1/2, Scope5/5
  Gateway Out/1 -> Add3/2, Scope5/2
  In2/1 -> Gateway Out/1
  In3/1 -> Gateway Out1/1
  In1/1 -> Unbuffer/1
  Unbuffer/1 -> Complex to Real-Imag/1

== system Basic_DMT/SIPaFFT/Assert_aft_FFT ==
  note: Das LSB wird unterschiedlich gerundet für 12 Nachkommastellen
  In1 : Inport
  In2 : Inport  Port=2
  In3 : Inport  Port=3
  Abs{,1..5} (6 alike) : Abs
  Add1 : Sum  Inputs=+-
  Add2 : Sum  Inputs=+-
  Add3 : Sum  Inputs=+-
  Check Static Range1 : simulink/Model Verification/Check  Static Range  Description=-1 <= u <= 1  max=1  max_included=on  min=-1  min_included=on  enabled=off  stopWhenAssertionFail=off  export=off  icon=graphic
  Check Static Range2 : simulink/Model Verification/Check  Static Range  Description=-1e-3 <= u <= 1e-3  max=1e-3  max_included=on  min=-1e-3  min_included=on  enabled=off  stopWhenAssertionFail=off  export=off  icon=graphic
  Check Static Range3 : simulink/Model Verification/Check  Static Range  Description=-1e-3 <= u <= 1e-3  max=1e-3  max_included=on  min=-1e-3  min_included=on  enabled=off  stopWhenAssertionFail=off  export=off  icon=graphic
  Complex to Real-Imag : ComplexToRealImag
  Data Type Conversion1 : DataTypeConversion  OutDataTypeStr=double
  Data Type Conversion2 : DataTypeConversion  OutDataTypeStr=double
  Delay : Delay  Commented=through  DelayLength=57  InitialCondition=0
  Divide : Product  Inputs=*/
  Divide1 : Product  Inputs=*/
  Divide2 : Product  Inputs=*/
  Gateway Out6 : xbsIndex_r4/Gateway Out  inherit_from_input=off  hdl_port=off  rows=1  columns=1  UseAsDAC=off  DACChannel='1'  interface=None  automatic_assignment=on  address_offset=hex2dec('00')  intf_description=''  timing_constraint=None  locs_specified=off  LOCs={}  io_standard={}  block_type=gatewayout
  Gateway Out7 : xbsIndex_r4/Gateway Out  inherit_from_input=off  hdl_port=off  rows=1  columns=1  UseAsDAC=off  DACChannel='1'  interface=None  automatic_assignment=on  address_offset=hex2dec('00')  intf_description=''  timing_constraint=None  locs_specified=off  LOCs={}  io_standard={}  block_type=gatewayout
  MinMax : MinMax  Function=max  Inputs=2
  MinMax1 : MinMax  Function=max  Inputs=2
  MinMax2 : MinMax  Function=max  Inputs=2
  Real-Imag to Complex : RealImagToComplex
  Reinterpret1 : xbsIndex_r4/Reinterpret  force_arith_type=on  arith_type="Signed  (2's comp)"  force_bin_pt=on  bin_pt=fracLen  block_type=reinterpret
  Reinterpret2 : xbsIndex_r4/Reinterpret  force_arith_type=on  arith_type="Signed  (2's comp)"  force_bin_pt=on  bin_pt=fracLen  block_type=reinterpret
  Scope1 : Scope  Commented=on  NumInputPorts=4
      settings: YMin=-5~-5~-5~-5  YMax=5~5~5~5  SaveName=ScopeData23
  Scope10 : Scope  NumInputPorts=4
      settings: YMin=-5~-5~-5~-5  YMax=5~5~5~5  SaveName=ScopeData20
  Scope3 : Scope  NumInputPorts=4
      settings: YMin=-5~-5~-5~-5  YMax=5~5~5~5  SaveName=ScopeData21
  Unbuffer : Unbuffer  SampleBasedProcessing=Same as frame based
  wires:
  Data Type Conversion2/1 -> Abs1/1
  Add1/1 -> Check Static Range3/1, Scope10/3, Divide/1
  In1/1 -> Unbuffer/1
  Complex to Real-Imag/1 -> Add1/1, Abs4/1, Scope10/1
  In3/1 -> Reinterpret1/1
  In2/1 -> Reinterpret2/1
  Abs/1 -> MinMax2/2, Add3/2, Scope1/2
  Add3/1 -> Divide2/1, Check Static Range2/1, Scope1/3
  Abs1/1 -> Scope1/1, MinMax2/1, Add3/1
  Gateway Out6/1 -> Real-Imag to Complex/1, Add1/2, Abs5/1, Scope10/2
  Data Type Conversion1/1 -> Abs/1
  Real-Imag to Complex/1 -> Data Type Conversion1/1
  Delay/1 -> Data Type Conversion2/1, Complex to Real-Imag/1
  MinMax/1 -> Divide/2
  Divide/1 -> Scope10/4
  Add2/1 -> Divide1/1, Check Static Range1/1, Scope3/3
  Complex to Real-Imag/2 -> Abs3/1, Scope3/1, Add2/1
  Gateway Out7/1 -> Real-Imag to Complex/2, Abs2/1, Scope3/2, Add2/2
  MinMax1/1 -> Divide1/2
  Divide1/1 -> Scope3/4
  Divide2/1 -> Scope1/4
  MinMax2/1 -> Divide2/2
  Unbuffer/1 -> Delay/1
  Reinterpret2/1 -> Gateway Out6/1
  Reinterpret1/1 -> Gateway Out7/1
  Abs2/1 -> MinMax1/2
  Abs3/1 -> MinMax1/1
  Abs4/1 -> MinMax/1
  Abs5/1 -> MinMax/2

== system Basic_DMT/SIPaFFT/Assert_bef_rem_GI ==
  In1 : Inport
  In2 : Inport  Port=2
  In3 : Inport  Port=3
  Add1 : Sum  Inputs=+-
  Add3 : Sum  Inputs=+-
  Check Static Range1 : simulink/Model Verification/Check  Static Range  Description=0 <= u <= 0  max=0  max_included=on  min=0  min_included=on  enabled=on  stopWhenAssertionFail=off  export=off  icon=graphic
  Check Static Range3 : simulink/Model Verification/Check  Static Range  Description=0 <= u <= 0  max=0  max_included=on  min=0  min_included=on  enabled=on  stopWhenAssertionFail=off  export=off  icon=graphic
  Complex to Real-Imag : ComplexToRealImag
  Gateway Out : xbsIndex_r4/Gateway Out  inherit_from_input=on  hdl_port=off  rows=1  columns=1  UseAsDAC=off  DACChannel='1'  interface=None  automatic_assignment=on  address_offset=hex2dec('00')  intf_description=''  timing_constraint=None  locs_specified=off  LOCs={}  io_standard={}  block_type=gatewayout
  Gateway Out1 : xbsIndex_r4/Gateway Out  inherit_from_input=on  hdl_port=off  rows=1  columns=1  UseAsDAC=off  DACChannel='1'  interface=None  automatic_assignment=on  address_offset=hex2dec('00')  intf_description=''  timing_constraint=None  locs_specified=off  LOCs={}  io_standard={}  block_type=gatewayout
  Scope5 : Scope  NumInputPorts=6
      settings: TimeRange=1.34597158739963e-06  YMin=-60~-60~-50~-20~-20~-50  YMax=20~20~50~60~60~50  SaveName=ScopeData18
  wires:
  Complex to Real-Imag/1 -> Scope5/1, Add3/1
  Add3/1 -> Check Static Range3/1, Scope5/3
  Complex to Real-Imag/2 -> Add1/1, Scope5/4
  Add1/1 -> Check Static Range1/1, Scope5/6
  Gateway Out1/1 -> Add1/2, Scope5/5
  Gateway Out/1 -> Add3/2, Scope5/2
  In2/1 -> Gateway Out/1
  In3/1 -> Gateway Out1/1
  In1/1 -> Complex to Real-Imag/1

== system Basic_DMT/SIPaFFT/Assert_rem_GI ==
  note: OFDM 24
  In1 : Inport
  In2 : Inport  Port=2
  In3 : Inport  Port=3
  before_GI : Inport  Port=4
  Add1 : Sum  Inputs=+-
  Add3 : Sum  Inputs=+-
  Check Static Range1 : simulink/Model Verification/Check  Static Range  Description=0 <= u <= 0  max=0  max_included=on  min=0  min_included=on  enabled=on  stopWhenAssertionFail=off  export=off  icon=graphic
  Check Static Range3 : simulink/Model Verification/Check  Static Range  Description=0 <= u <= 0  max=0  max_included=on  min=0  min_included=on  enabled=on  stopWhenAssertionFail=off  export=off  icon=graphic
  Complex to Real-Imag : ComplexToRealImag
  Complex to Real-Imag1 : ComplexToRealImag
  Delay : Delay  DelayLength=17+7+40  InitialCondition=0
  Gateway Out : xbsIndex_r4/Gateway Out  inherit_from_input=on  hdl_port=off  rows=1  columns=1  UseAsDAC=off  DACChannel='1'  interface=None  automatic_assignment=on  address_offset=hex2dec('00')  intf_description=''  timing_constraint=None  locs_specified=off  LOCs={}  io_standard={}  block_type=gatewayout
  Gateway Out1 : xbsIndex_r4/Gateway Out  inherit_from_input=on  hdl_port=off  rows=1  columns=1  UseAsDAC=off  DACChannel='1'  interface=None  automatic_assignment=on  address_offset=hex2dec('00')  intf_description=''  timing_constraint=None  locs_specified=off  LOCs={}  io_standard={}  block_type=gatewayout
  Scope5 : Scope  NumInputPorts=8
      settings: YMin=-5~-5~-5~-5~-5~-5~-5~-5  YMax=5~5~5~5~5~5~5~5  SaveName=ScopeData18
  Unbuffer : Unbuffer  SampleBasedProcessing=Same as frame based
  Unbuffer1 : Unbuffer  SampleBasedProcessing=Same as frame based
  wires:
  Complex to Real-Imag/1 -> Scope5/2, Add3/1
  Add3/1 -> Scope5/4, Check Static Range3/1
  Complex to Real-Imag/2 -> Scope5/6, Add1/1
  Add1/1 -> Scope5/8, Check Static Range1/1
  Gateway Out1/1 -> Scope5/7, Add1/2
  Gateway Out/1 -> Scope5/3, Add3/2
  In2/1 -> Gateway Out/1
  In3/1 -> Gateway Out1/1
  In1/1 -> Unbuffer/1
  Unbuffer/1 -> Complex to Real-Imag/1
  before_GI/1 -> Unbuffer1/1
  Complex to Real-Imag1/1 -> Scope5/1
  Complex to Real-Imag1/2 -> Scope5/5
  Unbuffer1/1 -> Delay/1
  Delay/1 -> Complex to Real-Imag1/1

== system Basic_DMT/SIPaFFT/Delay_Guard_Interval1 ==
  note: 1) Add Subsystem or Model blocks as valid variant choices.
      | 2) You cannot connect blocks at this level. At simulation, connectivity is automatically
      | determined, based on the active variant and port name matching.
  In1 : Inport
  None : Subsystem  VariantControl=guardInterval==1
  Rem_GI : Subsystem  VariantControl=guardInterval==2
  Out1 : Outport

== system Basic_DMT/SIPaFFT/Delay_Guard_Interval2 ==
  note: 1) Add Subsystem or Model blocks as valid variant choices.
      | 2) You cannot connect blocks at this level. At simulation, connectivity is automatically
      | determined, based on the active variant and port name matching.
  In1 : Inport
  In2 : Inport  Port=2
  In3 : Inport  Port=3
  In4 : Inport  Port=4
  In5 : Inport  Port=5
  In6 : Inport  Port=6
  In7 : Inport  Port=7
  In8 : Inport  Port=8
  In9 : Inport  Port=9
  In10 : Inport  Port=10
  In11 : Inport  Port=11
  In12 : Inport  Port=12
  In13 : Inport  Port=13
  In14 : Inport  Port=14
  In15 : Inport  Port=15
  In16 : Inport  Port=16
  No_equal : Subsystem  VariantControl=equalizer==1
  Yes_equal : Subsystem  VariantControl=equalizer==2
  Out1 : Outport
  Out2 : Outport  Port=2
  Out3 : Outport  Port=3
  Out4 : Outport  Port=4
  Out5 : Outport  Port=5
  Out6 : Outport  Port=6
  Out7 : Outport  Port=7
  Out8 : Outport  Port=8
  Out9 : Outport  Port=9
  Out10 : Outport  Port=10
  Out11 : Outport  Port=11
  Out12 : Outport  Port=12
  Out13 : Outport  Port=13
  Out14 : Outport  Port=14
  Out15 : Outport  Port=15
  Out16 : Outport  Port=16

== system Basic_DMT/SIPaFFT/Delay_upsample ==
  note: 1) Add Subsystem or Model blocks as valid variant choices.
      | 2) You cannot connect blocks at this level. At simulation, connectivity is automatically
      | determined, based on the active variant and port name matching.
  In1 : Inport
  Del_ups : Subsystem  VariantControl=upsample==2&&guardInterval==1
  Del_ups_GI : Subsystem  VariantControl=upsample==2&&guardInterval==2
  Delay_None : Subsystem  VariantControl=upsample==1
  Out1 : Outport

== system Basic_DMT/SIPaFFT/FFT ==
  note: 1) Add Subsystem or Model blocks as valid variant choices.
      | 2) You cannot connect blocks at this level. At simulation, connectivity is automatically
      | determined, based on the active variant and port name matching.
  In1 : Inport
  FFT_DMT : Subsystem  VariantControl=dmtOfdm==2
  FFT_OFDM : Subsystem  VariantControl=dmtOfdm==1
  Out1 : Outport
  db_aft_DMT : Outport  Port=2

== system Basic_DMT/SIPaFFT/Remove_Guard_Interval ==
  note: 1) Add Subsystem or Model blocks as valid variant choices.
      | 2) You cannot connect blocks at this level. At simulation, connectivity is automatically
      | determined, based on the active variant and port name matching.
  In1 : Inport
  No_GI : Subsystem  VariantControl=guardInterval==1
  Rem_GI_DMT : Subsystem  VariantControl=guardInterval==2&&dmtOfdm==2
  Rem_GI_OFDM : Subsystem  VariantControl=guardInterval==2&&dmtOfdm==1
  Out1 : Outport

== system Basic_DMT/SIPaFFT/downsample ==
  note: 1) Add Subsystem or Model blocks as valid variant choices.
      | 2) You cannot connect blocks at this level. At simulation, connectivity is automatically
      | determined, based on the active variant and port name matching.
  In1 : Inport
  No_downsample : Subsystem  VariantControl=upsample==1
  Yes_downsample : Subsystem  VariantControl=upsample==2
  Out1 : Outport

== system Basic_DMT/Sysgen_AWGN/No_AWGN ==
  Re : Inport
  Im : Inport  Port=2
  Constant : xbsIndex_r4/Constant  const=1  gui_display_data_type=Boolean  arith_type=Boolean  n_bits=16  bin_pt=14  preci_type=Single  exp_width=8  frac_width=24  explicit_period=off  period=1  equ=P=C  opselect=C  inp2=PCIN>>17  opr=+  inp1=P  carry=CIN  dbl_ovrd=off  block_type=constant
  Constant1 : xbsIndex_r4/Constant  const=1  gui_display_data_type=Fixed-point  arith_type=Signed (2's comp)  n_bits=bitCount+(log2(fftLen)+1)  bin_pt=fracLen  preci_type=Single  exp_width=8  frac_width=24  explicit_period=off  period=1  equ=P=C  opselect=C  inp2=PCIN>>17  opr=+  inp1=P  carry=CIN  dbl_ovrd=off  block_type=constant
  Re_out : Outport
  Im_out : Outport  Port=2
  db_bool : Outport  Port=3
  db_full : Outport  Port=4
  wires:
  Re/1 -> Re_out/1
  Im/1 -> Im_out/1
  Constant/1 -> db_bool/1
  Constant1/1 -> db_full/1
